simulink model "Observer_Reduced_model"  (R2015b)
settings: Solver=FixedStepAuto  StartTime=0.0  StopTime=30  FixedStep=Ts  MaxStep=0.005  RelTol=1e-3
InitFcn:
  | Ts=0.01;
values from neighbouring files (symbols this model uses):
  A = [-1/Tg1     0      -1/(R1*Tg1)   0       0       0        0 ... (first row only)    [ObserverModel_2area.m]
  B = [ 1/Tg1 0    0    0 ... (first row only)    [ObserverModel_2area.m]
  C = [0 0 B1  1 0 0 0 ... (first row only)    [ObserverModel_2area.m]
  dPL1 = 1    [ObserverModel_2area.m]
  dPL2 = 0    [ObserverModel_2area.m]
  L = place(A',C',Pole_obs)'    [ObserverModel_2area.m]
  Lred = place(a',c',Pole_redobs)'    [ObserverModel_2area.m]
undefined symbols (not defined in the file or in its folder): a, b, c, T
settings Model: Creator=Majidi  LastModifiedBy=Admin
settings DataIOCC: SaveFormat=Array
settings OptimizationCC: ExpressionDepthLimit=2147483647
settings DebuggingCC: UnderspecifiedInitializationDetection=Classic  MergeDetectMultiDrivingBlocksExec=none  SolverPrmCheckMsg=warning  StateNameClashWarn=warning
settings HardwareCC: ProdBitPerPointer=32  ProdLargestAtomicFloat=None  ProdIntDivRoundTo=Undefined  ProdEndianess=Unspecified  ProdWordSize=32  ProdHWDeviceType=32-bit Generic
settings GRTTargetCC: GeneratePreprocessorConditionals=Disable all
settings ConfigComp: CovModelRefEnable=Off

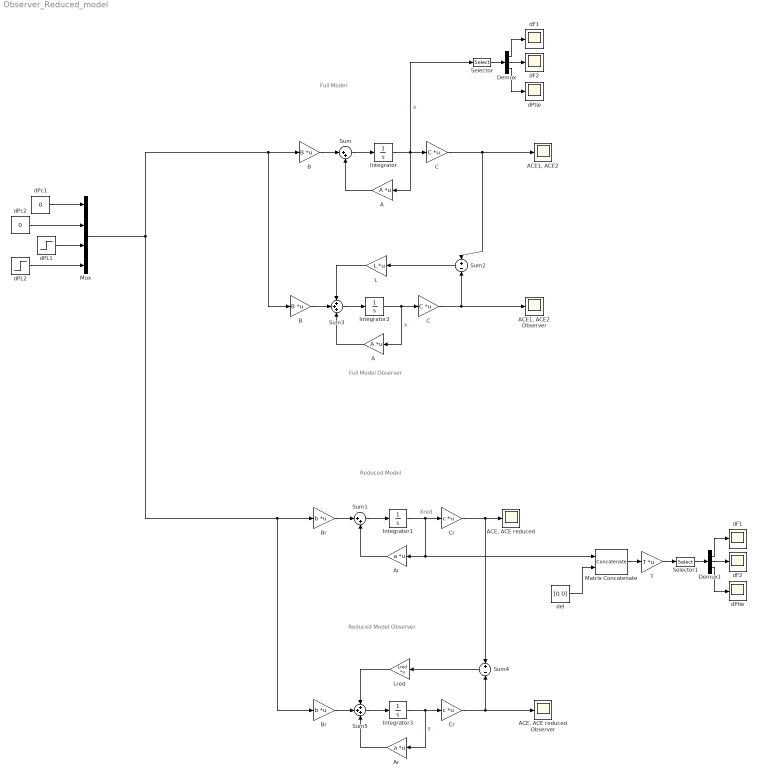
== system Observer_Reduced_model ==
  note: Reduced Model
  note: Xred
  note: Full Model
  note: Full Model Observer
  note: Reduced Model Observer
  A : Gain  Gain=A  Multiplication=Matrix(K*u)
  "A " : Gain  Gain=A  Multiplication=Matrix(K*u)
  "ACE, ACE reduced" : Scope
  "ACE, ACE reduced Observer" : Scope
  "ACE1, ACE2" : Scope
  "ACE1, ACE2 Observer" : Scope
  Ar : Gain  Gain=a  Multiplication=Matrix(K*u)
  "Ar " : Gain  Gain=a  Multiplication=Matrix(K*u)
  B : Gain  Gain=B  Multiplication=Matrix(K*u)
  "B " : Gain  Gain=B  Multiplication=Matrix(K*u)
  Br : Gain  Gain=b  Multiplication=Matrix(K*u)
  "Br " : Gain  Gain=b  Multiplication=Matrix(K*u)
  C : Gain  Gain=C  Multiplication=Matrix(K*u)
  "C " : Gain  Gain=C  Multiplication=Matrix(K*u)
  Cr : Gain  Gain=c  Multiplication=Matrix(K*u)
  "Cr " : Gain  Gain=c  Multiplication=Matrix(K*u)
  Demux : Demux  Outputs=3
  Demux1 : Demux  Outputs=3
  Integrator : Integrator
  Integrator1 : Integrator
  Integrator2 : Integrator  InitialCondition=[0 0 1 0 0 0 1]
  Integrator3 : Integrator  InitialCondition=[1 0 0 0 0]
  L : Gain  Gain=L  Multiplication=Matrix(K*u)
  Lred : Gain  Gain=Lred  Multiplication=Matrix(K*u)
  Matrix Concatenate : Concatenate  ConcatenateDimension=2
  Mux : Mux
  Selector : Selector  InputPortWidth=7  IndexOptions=Index vector (dialog)  Indices=[3 4 7]  OutputSizes=1
  Selector1 : Selector  InputPortWidth=7  IndexOptions=Index vector (dialog)  Indices=[3 4 7]  OutputSizes=1
  Sum : Sum  Inputs=|++
  Sum1 : Sum  Inputs=|++
  Sum2 : Sum  Inputs=+|-
  Sum3 : Sum  Inputs=+++
  Sum4 : Sum  Inputs=+|-
  Sum5 : Sum  Inputs=+++
  "T " : Gain  Gain=T  Multiplication=Matrix(K*u)
  dF1 : Scope
  "dF1 " : Scope
  dF2 : Scope
  "dF2 " : Scope
  dPL1 : Step  After=dPL1  SampleTime=0
  dPL2 : Step  After=dPL2  SampleTime=0
  dPc1 : Constant  Value=0
  dPc2 : Constant  Value=0
  dPtie : Scope
  "dPtie " : Scope
  del : Constant  Value=[0 0]
  wires:
  B/1 -> Sum/1
  Sum/1 -> Integrator/1
  A/1 -> Sum/2
  Integrator/1 -> Selector/1, A/1, C/1  "X"
  C/1 -> "ACE1, ACE2"/1, Sum2/1
  dPL1/1 -> Mux/3
  dPL2/1 -> Mux/4
  dPc1/1 -> Mux/1
  dPc2/1 -> Mux/2
  Demux/1 -> dF1/1
  Demux/2 -> dF2/1
  Demux/3 -> dPtie/1
  Selector/1 -> Demux/1
  Br/1 -> Sum1/1
  Sum1/1 -> Integrator1/1
  Ar/1 -> Sum1/2
  Integrator1/1 -> Cr/1, Ar/1, Matrix Concatenate/1
  Mux/1 -> B/1, "B "/1, "Br "/1, Br/1
  Cr/1 -> "ACE, ACE reduced"/1, Sum4/1
  del/1 -> Matrix Concatenate/2
  Matrix Concatenate/1 -> "T "/1
  "T "/1 -> Selector1/1
  Demux1/1 -> "dF1 "/1
  Demux1/2 -> "dF2 "/1
  Demux1/3 -> "dPtie "/1
  Selector1/1 -> Demux1/1
  "B "/1 -> Sum3/2
  Sum3/1 -> Integrator2/1
  "A "/1 -> Sum3/3
  Integrator2/1 -> "C "/1, "A "/1  "X"
  "C "/1 -> "ACE1, ACE2 Observer"/1, Sum2/2
  Sum2/1 -> L/1
  L/1 -> Sum3/1
  "Br "/1 -> Sum5/2
  Sum5/1 -> Integrator3/1
  "Ar "/1 -> Sum5/3
  Integrator3/1 -> "Ar "/1, "Cr "/1  "X"
  Sum4/1 -> Lred/1
  Lred/1 -> Sum5/1
  "Cr "/1 -> "ACE, ACE reduced Observer"/1, Sum4/2
